simulink subsystem "protect_rotation"  (R2021a)
settings: Solver=VariableStepAuto  StartTime=0.0  StopTime=10.0  RelTol=1e-3
values from neighbouring files (symbols this model uses):
  angle_limit : value not decoded    [common_data.sldd]
  init_time = 1.0    [common_data.sldd]
settings Model: Creator=tshintai  LastModifiedBy=tshintai

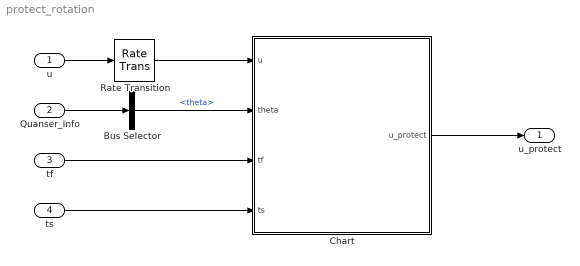
== system protect_rotation ==
  u : Inport
  Quanser_Info : Inport  Port=2
  tf : Inport  Port=3
  ts : Inport  Port=4
  Bus Selector : BusSelector  OutputSignals=theta
  Chart : Stateflow chart  TreatAsAtomicUnit=on
  Rate Transition : RateTransition  OutPortSampleTime=ts_raspi
  u_protect : Outport
  wires:
  Rate Transition/1 -> Chart/1(u)
  Chart/1(u_protect) -> u_protect/1
  Bus Selector/1 -> Chart/2(theta)  "<theta>"
  Quanser_Info/1 -> Bus Selector/1
  u/1 -> Rate Transition/1
  tf/1 -> Chart/3(tf)
  ts/1 -> Chart/4(ts)

== stateflow chart protect_rotation/Chart ==
  state StandBy
    entry:
    u_protect = 0;
    during:
    u_protect = 0;
  state Normal
    entry:
    u_protect = u;
    during:
    u_protect = u;
  state Terminate
    entry:
    u_protect = 0;
    during:
    u_protect = 0;
  state Emergency
    entry:
    u_protect = 0;
    during:
    u_protect = 0;
  (default) -> StandBy
  StandBy -> Normal : [
      | after(init_time, sec)
      | ]
  Normal -> Terminate [order 2] : [
      | after(tf - ts -init_time, sec)
      | ]
  Normal -> Emergency [order 1] : [
      | abs(theta) >= angle_limit
      | ]
  data: u input; theta input; u_protect output; angle_limit parameter; init_time parameter; tf input; ts input
